simulink model "kuka_simulink_control"  (R2013b)
settings: Solver=FixedStepDiscrete  StartTime=0.0  StopTime=inf  FixedStep=0.01  RelTol=1e-3
StartFcn:
  | jankov_var = 10;
libraries: robotica x1
settings Model: Creator=jankokolar  LastModifiedBy=student
settings DebuggingCC: StateNameClashWarn=warning

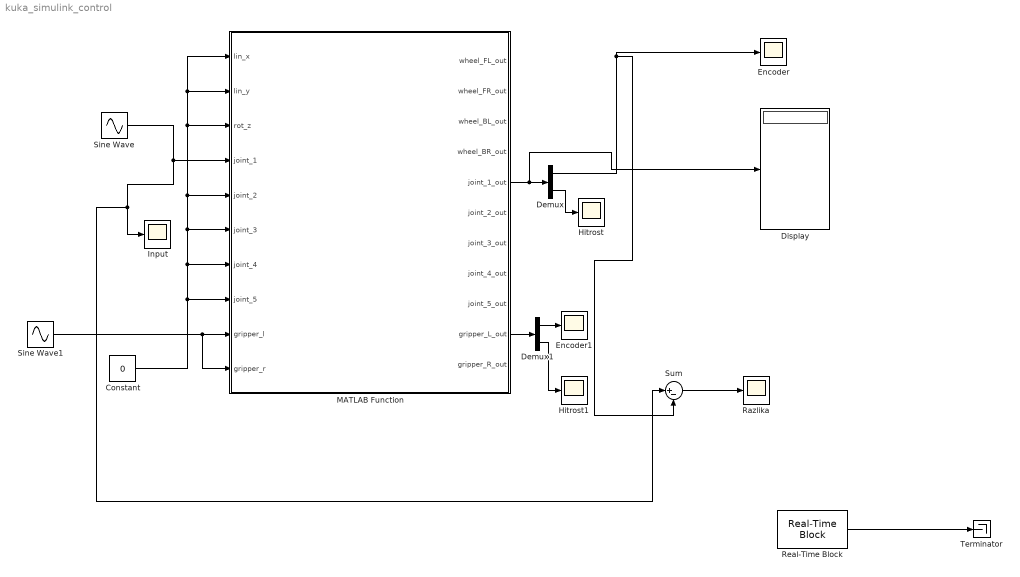
== system kuka_simulink_control ==
  Constant : Constant  Value=0
  Demux : Demux  Outputs=2
  Demux1 : Demux  Outputs=2
  Display : Display
  Encoder : Scope
      settings: YMin=2.77556e-17  YMax=1.05
  Encoder1 : Scope
      settings: YMin=6.09848e-06  YMax=6.09848e-06  SaveName=ScopeData4
  Hitrost : Scope
      settings: YMin=-0.25  YMax=0.4  SaveName=ScopeData3
  Hitrost1 : Scope
      settings: YMin=-0.25  YMax=0.4  SaveName=ScopeData5
  Input : Scope
      settings: YMin=0.75  YMax=1.025
  MATLAB Function : MATLAB Function  StartFcn=|  StopFcn=|  TreatAsAtomicUnit=on
      StartFcn=|
      | ros_node = rosmatlab.node('KUKA_SIMULINK_CONTROL','192.168.65.59',11311);          
      | 
      | % Base                                        
      | 
      |     publisher_na_kuko = rosmatlab.publisher('/cmd_vel','geometry_msgs/Twist',ros_node);                                     
      |     kuka_message = rosmatlab.message('geometry_msgs/Twist',ros_node);                                                       
      |     kuka_message.getLinear.setX(0.0);                                                                                       
      |     kuka_message.getLinear.setY(0);                                                                                         
      |     kuka_message.getLinear.setZ(0);                                                                                         
      |     kuka_message.getAngular.setX(0);                                                                                        
      |     kuka_message.getAngular.setY(0);                                                                                        
      |     kuka_message.getAngular.setZ(0);                                                                                        
      |     publisher_na_kuko.publish(kuka_message);                                                                                
      | 
      | % Arm
      |                                                                                                                             
      | publisher_kuka_arm = rosmatlab.publisher('/arm_1/arm_controller/position_command','brics_actuator/JointPositions',ros_node);
      |                                                                                                                             
      | arm_kuka_message = rosmatlab.message('brics_actuator/JointPositions', ros_node);                                            
      |                                                                                                                             
      | arm_header_message = rosmatlab.message('brics_actuator/Poison', ros_node);                                                  
      |                                                                                                                             
      | joint_1_message =  rosmatlab.message('brics_actuator/JointValue', ros_node);                                                
      |                                                                                                                             
      | joint_2_message= rosmatlab.message('brics_actuator/JointValue', ros_node);                                                  
      |                                                                                                                             
      | joint_3_message = rosmatlab.message('brics_actuator/JointValue', ros_node);                                                 
      |                                                                                                                             
      | joint_4_message = rosmatlab.message('brics_actuator/JointValue', ros_node);                                                 
      |                                                                                                                             
      | joint_5_message = rosmatlab.message('brics_actuator/JointValue', ros_node);                                                 
      |                                                                                                                             
      | arm_header_message.setDescription('Pozdrav iz Simulinka');                                                                  
      | arm_header_message.setOriginator('Simulink');                                                                               
      | arm_header_message.setQos(0.0);                                                                                             
      | arm_kuka_message.setPoisonStamp(arm_header_message);                                                                        
      |                                                                                                                             
      | joint_1_message.setJointUri('arm_joint_1');                                                                                 
      | joint_1_message.setUnit('rad');                                                                                             
      | joint_1_message.setValue(0.02);                                                                                                
      |                                                                                                                             
      | joint_2_message.setJointUri('arm_joint_2');                                                                                 
      | joint_2_message.setUnit('rad');                                                                                             
      | joint_2_message.setValue(0.02);                                                                                                
      |                                                                                                                             
      | joint_3_message.setJointUri('arm_joint_3');                                                                                 
      | joint_3_message.setUnit('rad');                                                                                             
      | joint_3_message.setValue(-0.02);                                                                                                
      |                                                                                                                             
      | joint_4_message.setJointUri('arm_joint_4');                                                                                 
      | joint_4_message.setUnit('rad');                                                                                             
      | joint_4_message.setValue(0.023);                                                                                                
      |                                                                                                                             
      | joint_5_message.setJointUri('arm_joint_5');                                                                                 
      | joint_5_message.setUnit('rad');                                                                                             
      | joint_5_message.setValue(0.12);                                                                                                
      |                                                                                                                             
      | arm_kuka_message.getPositions.add(joint_1_message);                                                                         
      | arm_kuka_message.getPositions.add(joint_2_message);                                                                         
      | arm_kuka_message.getPositions.add(joint_3_message);                                                                         
      | arm_kuka_message.getPositions.add(joint_4_message);                                                                         
      | arm_kuka_message.getPositions.add(joint_5_message);                                                                         
      |                                                                                                                             
      | publisher_kuka_arm.publish(arm_kuka_message);     
      | 
      | % Gripper
      | 
      | gripper_publisher = rosmatlab.publisher('/arm_1/gripper_controller/position_command','brics_actuator/JointPositions',ros_node);
      | 
      | gripper_message = rosmatlab.message('brics_actuator/JointPositions', ros_node);
      | gripper_header_message = rosmatlab.message('brics_actuator/Poison', ros_node);
      | gripper_L_message =  rosmatlab.message('brics_actuator/JointValue', ros_node);
      | gripper_R_message= rosmatlab.message('brics_actuator/JointValue', ros_node);
      | 
      | gripper_header_message.setDescription('Hello Simulink.  Gripper greets you');
      | gripper_header_message.setOriginator('Simulink');
      | gripper_header_message.setQos(0.0);
      | gripper_message.setPoisonStamp(gripper_header_message);
      | 
      | gripper_L_message.setJointUri('gripper_finger_joint_l');
      | gripper_L_message.setUnit('m');
      | gripper_L_message.setValue(0);
      | 
      | gripper_R_message.setJointUri('gripper_finger_joint_r');
      | gripper_R_message.setUnit('m');
      | gripper_R_message.setValue(0);
      | 
      | gripper_message.getPositions.add(gripper_L_message);
      | gripper_message.getPositions.add(gripper_R_message);
      | 
      | gripper_publisher.publish(gripper_message);
      |   
      | % assign reader
      | arm_position = zeros(7,1);
      | arm_velocities = zeros(7,1);
      | 
      | base_position = zeros(8,1);
      | base_velocities = zeros(8,1);
      |            
      | encoder_reader = rosmatlab.subscriber('/joint_states','sensor_msgs/JointState',10,ros_node);
      | 
      | encoder_reader.setOnNewMessageListeners({@read_encoders})
      StopFcn=|
      | kuka_message.getLinear.setX(0);         
      | kuka_message.getLinear.setY(0);         
      | kuka_message.getLinear.setZ(0);         
      | kuka_message.getAngular.setX(0);        
      | kuka_message.getAngular.setY(0);        
      | kuka_message.getAngular.setZ(0);        
      | publisher_na_kuko.publish(kuka_message);
      | encoder_reader.setOnNewMessageListeners({[]})          
      | ros_node.delete                         
      | clear all
  Razlika : Scope
      settings: YMin=-0.08  YMax=0.06  SaveName=ScopeData2
  Real-Time Block : robotica/Utilities blocks/Real-Time Block  sync_type=Fixed  sync_time=0.01
  Sine Wave : Sin  Amplitude=0.5  Bias=0.52  Frequency=0.5  Phase=-3.1415/2  SampleTime=0
  Sine Wave1 : Sin  Amplitude=0.005  Bias=0.005  Frequency=0.5  Phase=-3.1415/2  SampleTime=0
  Sum : Sum  Inputs=|+-
  Terminator : Terminator
  wires:
  Real-Time Block/1 -> Terminator/1
  Constant/1 -> MATLAB Function/5(joint_2), MATLAB Function/3(rot_z), MATLAB Function/2(lin_y), MATLAB Function/1(lin_x), MATLAB Function/6(joint_3), MATLAB Function/7(joint_4), MATLAB Function/8(joint_5)
  Demux/1 -> Encoder/1, Sum/2
  Sum/1 -> Razlika/1
  Sine Wave/1 -> MATLAB Function/4(joint_1), Sum/1, Input/1
  MATLAB Function/5(joint_1_out) -> Display/1, Demux/1
  Demux/2 -> Hitrost/1
  Sine Wave1/1 -> MATLAB Function/10(gripper_r), MATLAB Function/9(gripper_l)
  MATLAB Function/10(gripper_L_out) -> Demux1/1
  Demux1/1 -> Encoder1/1
  Demux1/2 -> Hitrost1/1

== matlab function kuka_simulink_control/MATLAB Function ==
  data: wheel_FL_out output; lin_x input; lin_y input; rot_z input; joint_1 input; joint_2 input; joint_3 input; joint_4 input; joint_5 input; gripper_l input; gripper_r input; wheel_FR_out output; wheel_BL_out output; wheel_BR_out output; joint_1_out output; joint_2_out output; joint_3_out output; joint_4_out output; joint_5_out output; gripper_L_out output; gripper_R_out output
function [wheel_FL_out,wheel_FR_out,wheel_BL_out,wheel_BR_out,joint_1_out, joint_2_out,joint_3_out,joint_4_out,joint_5_out,gripper_L_out, gripper_R_out] = kontrola_kuke(lin_x,lin_y,rot_z,joint_1,joint_2,joint_3,joint_4,joint_5,gripper_l,gripper_r)

persistent lin_x_old lin_y_old rot_z_old;
persistent joint_1_old joint_2_old joint_3_old joint_4_old joint_5_old ;
persistent gripper_l_old gripper_r_old ; 

if isempty(lin_x_old)  % all initialized at first step
    lin_x_old = 0;
    lin_y_old = 0;
    rot_z_old = 0;
    joint_1_old = 0;
    joint_2_old = 0;
    joint_3_old = 0 ;
    joint_4_old = 0;
    joint_5_old = 0; 
    gripper_l_old = 0;
    gripper_r_old = 0;
    
end

coder.extrinsic('num2str','strcat','evalin');

if lin_x ~= lin_x_old
    ukaz= strcat('kuka_message.getLinear.setX(',num2str(lin_x),')');
    evalin('base', ukaz);
end

if lin_y ~= lin_y_old
    ukaz= strcat('kuka_message.getLinear.setY(',num2str(lin_y),')');
    evalin('base', ukaz);
end

if rot_z ~= rot_z_old
    ukaz= strcat('kuka_message.getAngular.setZ(',num2str(rot_z),')');
    evalin('base', ukaz);
end

if (lin_x ~= lin_x_old)||(lin_y ~= lin_y_old)||(rot_z ~= rot_z_old)
    evalin('base','publisher_na_kuko.publish(kuka_message)');
end

if joint_1 ~= joint_1_old
    ukaz= strcat('joint_1_message.setValue(',num2str(joint_1),')');
    evalin('base', ukaz);
end

if joint_2 ~= joint_2_old
    ukaz= strcat('joint_2_message.setValue(',num2str(joint_2),')');
    evalin('base', ukaz);
end

if joint_3 ~= joint_3_old
    ukaz= strcat('joint_3_message.setValue(',num2str(joint_3),')');
    evalin('base', ukaz);
end

if joint_4 ~= joint_4_old
    ukaz= strcat('joint_4_message.setValue(',num2str(joint_4),')');
    evalin('base', ukaz);
end

if joint_5 ~= joint_5_old
    ukaz= strcat('joint_5_message.setValue(',num2str(joint_5),')');
    evalin('base', ukaz);
end

if (joint_1 ~= joint_1_old)||(joint_2 ~= joint_2_old)||(joint_3 ~= joint_3_old)||(joint_4 ~= joint_4_old)||(joint_5 ~= joint_5_old)
    evalin('base','publisher_kuka_arm.publish(arm_kuka_message)');
end

if gripper_l ~= gripper_l_old
    ukaz= strcat('gripper_L_message.setValue(',num2str(gripper_l),')');
    evalin('base', ukaz);
end

if gripper_r ~= gripper_r_old
    ukaz= strcat('gripper_R_message.setValue(',num2str(gripper_r),')');
    evalin('base', ukaz);
end

if (gripper_l ~= gripper_l_old)||(gripper_r ~= gripper_r_old)
    evalin('base','gripper_publisher.publish(gripper_message)');
end


lin_x_old = lin_x;
lin_y_old = lin_y;
rot_z_old = rot_z;
joint_1_old = joint_1;
joint_2_old = joint_2;
joint_3_old = joint_3;
joint_4_old = joint_4;
joint_5_old = joint_5;
gripper_l_old = gripper_l;
gripper_r_old = gripper_r;

joint_positions = zeros(7,1);
joint_speeds = zeros(7,1);
joint_positions = evalin('base','arm_position');
joint_speeds = evalin('base','arm_velocities');

base_positions = zeros(8,1);
base_speeds = zeros(8,1);
base_positions = evalin('base','base_position');
base_speeds = evalin('base','base_velocities');

joint_1_out = [joint_positions(1); joint_speeds(1)];
joint_2_out = [joint_positions(2); joint_speeds(2)];
joint_3_out = [joint_positions(3); joint_speeds(3)];
joint_4_out = [joint_positions(4); joint_speeds(4)];
joint_5_out = [joint_positions(5); joint_speeds(5)];
gripper_L_out = [joint_positions(6); joint_speeds(6)];
gripper_R_out = [joint_positions(7); joint_speeds(7)];

wheel_FL_out = [base_positions(1); base_speeds(1)];
wheel_FR_out = [base_positions(2); base_speeds(2)];
wheel_BL_out = [base_positions(3); base_speeds(3)];
wheel_BR_out = [base_positions(4); base_speeds(4)];
